simulink model "simulink_paper"  (R2016a)
settings: Solver=FixedStepAuto  StartTime=0.0  StopTime=10.0  FixedStep=0.001  RelTol=1e-3
settings Model: Creator=Florian  LastModifiedBy=Florian

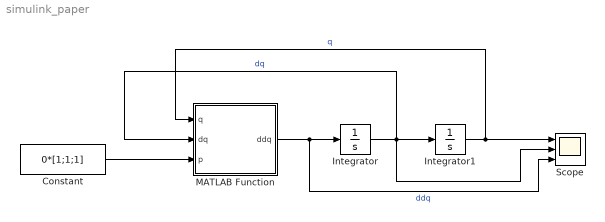
== system simulink_paper ==
  Constant : Constant  Value=0*[1;1;1]
  Integrator : Integrator  InitialCondition=[0;0;0]
  Integrator1 : Integrator  InitialCondition=[0.16; 0.16; 0.16]
  MATLAB Function : MATLAB Function  TreatAsAtomicUnit=on
  Scope : Scope  NumInputPorts=3
  wires:
  Integrator/1 -> Integrator1/1, Scope/2, MATLAB Function/2(dq)  "dq"
  Integrator1/1 -> Scope/1, MATLAB Function/1(q)  "q"
  MATLAB Function/1(ddq) -> Scope/3, Integrator/1  "ddq"
  Constant/1 -> MATLAB Function/3(p)

== matlab function simulink_paper/MATLAB Function ==
  data: q input; ddq output; dq input; p input
function ddq = fcn(q, dq, p)
%#codegen

if abs(q(1)-q(2)) < 0.0001 && abs(q(2)-q(3)) < 0.0001 && abs(q(1)-q(3)) < 0.0001
    invM = inv(Mfunc2(q));
    Q = Qfunc2(q, p);
    N = Nfunc2(q, dq);
else
    invM = inv(Mfunc(q));
    Q = Qfunc(q, p);
    N = Nfunc(q, dq);
end


ddq = invM * (Q - N);
